simulink model "Likitha_Version_4"  (R2025b)
settings: Solver=VariableStepAuto  StartTime=0.0  StopTime=0.3  RelTol=1e-3
undefined symbols (not defined in the file): Ion, Lithium
libraries: spsBatteryLib x50, spsSeriesRLCBranchLib x15, spsCurrentMeasurementLib x10, spsVoltageMeasurementLib x10, spsIdealSwitchLib x9, spsMosfetLib x7, slpidlib x4, spsPWMGeneratorDCDCLib x2, spspowerguiLib x2, spsACVoltageSourceLib x1, eeHysteresisControl x1, spsDCMachineLib x1
(part 4 of 4)

== matlab function Likitha_Version_4/Subsystem3/MATLAB Function ==
  data: SOC input; trainingData output; SOH input; SOP input; DOD input; ROH input; RUL input; CycleCount input; V_avg input; I_avg input; P_avg input; stress_idx input; aging_rate_frac input; energy_kWh input; degrad_idx input; T_idx input; health_idx input; I_peak input; V_min input; T_max input; Ah_charge_total input; Ah_discharge_total input; overtime_sec input; timestamp input; windowSize input; stepSize input; validationData output; features output; labels output; timeWindows output
function [trainingData, validationData, features, labels, timeWindows] = PreTrainingDataPrep(...
    SOC, SOH, SOP, DOD, ROH, RUL, CycleCount, ...
    V_avg, I_avg, P_avg, stress_idx, aging_rate_frac, energy_kWh, ...
    degrad_idx, T_idx, health_idx, I_peak, V_min, T_max, ...
    Ah_charge_total, Ah_discharge_total, overtime_sec, ...
    timestamp, windowSize, stepSize)
% PreTrainingDataPrep - Prepares data for AI/ML/DL model training
% 
% Inputs:
%   All 22 parameters from your second block
%   timestamp   : Current simulation time (s)
%   windowSize  : Size of sliding window for sequence data (e.g., 100 samples)
%   stepSize    : Step size for sliding window (e.g., 10 samples)
%
% Outputs:
%   trainingData    : Structure containing training datasets for different models
%   validationData  : Structure containing validation datasets
%   features        : Engineered features for ML models
%   labels          : Target labels for supervised learning
%   timeWindows     : Cell array of time-series windows for DL models

% -------------------------------------------------------------------------
% Persistent storage for historical data
% -------------------------------------------------------------------------
persistent paramHistory timestampHistory bufferIdx maxBufferSize
persistent windowedData windowLabels windowTimestamps

% Initialize on first call
if isempty(paramHistory)
    maxBufferSize = 10000;  % Store last 10,000 samples
    paramHistory = zeros(maxBufferSize, 22);  % 22 parameters
    timestampHistory = zeros(maxBufferSize, 1);
    bufferIdx = 1;
    
    % For windowing
    windowedData = {};
    windowLabels = {};
    windowTimestamps = {};
end

% -------------------------------------------------------------------------
% 1. Collect current sample into circular buffer
% -------------------------------------------------------------------------
currentParams = [SOC, SOH, SOP, DOD, ROH, RUL, CycleCount, ...
                 V_avg, I_avg, P_avg, stress_idx, aging_rate_frac, energy_kWh, ...
                 degrad_idx, T_idx, health_idx, I_peak, V_min, T_max, ...
                 Ah_charge_total, Ah_discharge_total, overtime_sec];

paramHistory(bufferIdx, :) = currentParams;
timestampHistory(bufferIdx) = timestamp;
bufferIdx = mod(bufferIdx, maxBufferSize) + 1;

% -------------------------------------------------------------------------
% 2. Extract non-overlapping windows for training when enough data accumulated
% -------------------------------------------------------------------------
if mod(timestamp, stepSize * 0.1) < 1e-6  % Check at each step size interval
    % Get valid contiguous data (handle buffer wrap-around)
    if bufferIdx > windowSize
        validHistory = paramHistory(1:bufferIdx-1, :);
        validTimestamps = timestampHistory(1:bufferIdx-1);
    else
        % Handle circular buffer wrap (simplified - use latest contiguous segment)
        validHistory = paramHistory(max(1, end-windowSize+1):end, :);
        validTimestamps = timestampHistory(max(1, end-windowSize+1):end);
    end
    
    % Create windows if we have enough data
    if size(validHistory, 1) >= windowSize
        numWindows = floor((size(validHistory, 1) - windowSize) / stepSize) + 1;
        
        for w = 1:numWindows
            startIdx = (w-1) * stepSize + 1;
            endIdx = startIdx + windowSize - 1;
            
            % Extract window data
            windowData = validHistory(startIdx:endIdx, :);
            windowTime = validTimestamps(startIdx:endIdx);
            
            % Store window
            windowedData{end+1} = windowData;
            windowTimestamps{end+1} = windowTime;
            
            % Generate labels based on future values (for prediction tasks)
            if endIdx + 10 <= size(validHistory, 1)  % Predict 10 steps ahead
                futureSOC = validHistory(endIdx + 10, 1);  % SOC is first column
                futureSOH = validHistory(endIdx + 10, 2);  % SOH is second column
                windowLabels{end+1} = [futureSOC, futureSOH];
            else
                windowLabels{end+1} = [windowData(end, 1), windowData(end, 2)];  % Use last values
            end
        end
    end
end

% -------------------------------------------------------------------------
% 3. Feature Engineering for Classical ML
% -------------------------------------------------------------------------
% Extract statistical features from the last window
if ~isempty(windowedData)
    latestWindow = windowedData{end};
    
    % Features for each parameter (22 parameters × 6 features = 132 features)
    features = [];
    for p = 1:22
        features = [features, ...
                    mean(latestWindow(:, p)), ...      % Mean
                    std(latestWindow(:, p)), ...       % Standard deviation
                    min(latestWindow(:, p)), ...       % Minimum
                    max(latestWindow(:, p)), ...       % Maximum
                    latestWindow(end, p) - latestWindow(1, p), ...  % Trend (delta)
                    sum(diff(latestWindow(:, p)) > 0)];  % Number of increases
    end
    
    % Add rate-of-change features
    if size(latestWindow, 1) > 1
        dt_window = mean(diff(windowTimestamps{end}));
        if dt_window > 0
            roc = diff(latestWindow) / dt_window;
            features = [features, mean(roc, 1), std(roc, 0, 1)];
        end
    end
    
    % Labels (targets for supervised learning)
    labels = windowLabels{end};
else
    features = zeros(1, 132 + 44);  % Placeholder
    labels = [SOC, SOH];
end

% -------------------------------------------------------------------------
% 4. Prepare training/validation datasets
% -------------------------------------------------------------------------
% Split data into training (70%) and validation (30%)
numWindows = length(windowedData);
if numWindows > 10
    splitIdx = round(0.7 * numWindows);
    
    % For time-series models (LSTM, Transformer) - keep temporal order
    trainingData.sequences = windowedData(1:splitIdx);
    trainingData.labels = windowLabels(1:splitIdx);
    trainingData.timestamps = windowTimestamps(1:splitIdx);
    
    validationData.sequences = windowedData(splitIdx+1:end);
    validationData.labels = windowLabels(splitIdx+1:end);
    validationData.timestamps = windowTimestamps(splitIdx+1:end);
    
    % For classical ML - flatten features
    trainingData.features = [];  % Would need to recompute features for each window
    validationData.features = [];
else
    trainingData = struct();
    validationData = struct();
end

% -------------------------------------------------------------------------
% 5. Add metadata for different model types
% -------------------------------------------------------------------------
trainingData.parameterNames = {'SOC', 'SOH', 'SOP', 'DOD', 'ROH', 'RUL', 'CycleCount', ...
                               'V_avg', 'I_avg', 'P_avg', 'stress_idx', 'aging_rate_frac', 'energy_kWh', ...
                               'degrad_idx', 'T_idx', 'health_idx', 'I_peak', 'V_min', 'T_max', ...
                               'Ah_charge_total', 'Ah_discharge_total', 'overtime_sec'};
trainingData.windowSize = windowSize;
trainingData.stepSize = stepSize;
trainingData.sampleRate = 1/mean(diff(timestampHistory(timestampHistory > 0)));

% Outputs
timeWindows = windowedData;

end
